simulink model "tutorial4"  (R2020a)
settings: Solver=FixedStepAuto  StartTime=0.0  StopTime=10.0  FixedStep=1e-3  RelTol=1e-3  EnableMultiTasking=on
libraries: dspstat3 x2
settings Model: ExtModeTrigDuration=5  Creator=qasim  LastModifiedBy=qasim
settings OptimizationCC: EnhancedBackFolding=on  PassReuseOutputArgsAs=Individual arguments  ZeroExternalMemoryAtStartup=off  ZeroInternalMemoryAtStartup=off  MaxStackSize=64  OptimizeBlockOrder=speed  DifferentSizesBufferReuse=on  OptimizationCustomize=off  EfficientTunableParamExpr=on
settings DebuggingCC: ParameterTunabilityLossMsg=error
settings HardwareCC: ProdBitPerPointer=32  ProdBitPerSizeT=32  ProdBitPerPtrDiffT=32  ProdLargestAtomicInteger=Long  ProdLargestAtomicFloat=Double  ProdWordSize=32  ProdHWDeviceType=ARM Compatible->ARM Cortex
settings SFSimCC: MATLABDynamicMemAlloc=off
settings RTWCC: SystemTargetFile=ert.tlc  HardwareBoard=NXP FRDM-K64F  TemplateMakefile=ert_default_tmf  Toolchain=GNU Tools for ARM Embedded Processors
settings CodeAppCC: ForceParamTrailComments=on  IgnoreCustomStorageClasses=off  OperatorAnnotations=on  SimulinkDataObjDesc=on  SFDataObjDesc=on  InsertBlockDesc=on

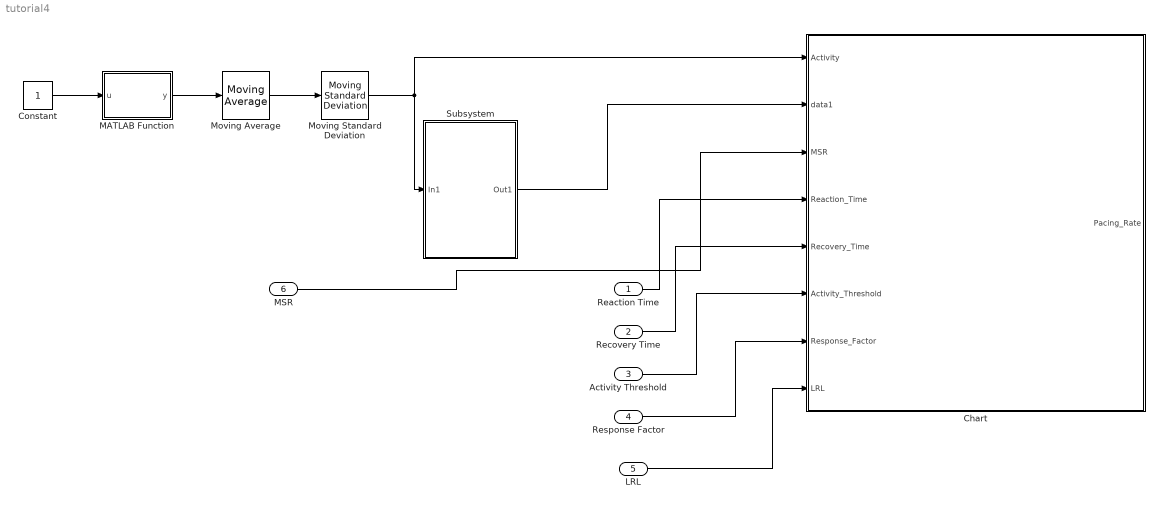
== system tutorial4 ==
  Reaction Time : Inport
  Recovery Time : Inport  Port=2
  Activity Threshold : Inport  Port=3
  Response Factor : Inport  Port=4
  LRL : Inport  Port=5
  MSR : Inport  Port=6
  Chart : Stateflow chart  TreatAsAtomicUnit=on
  Constant : Constant
  MATLAB Function : MATLAB Function  TreatAsAtomicUnit=on
  Moving Average : dspstat3/Moving Average  Method=Sliding window  ForgettingFactorPort=off  SpecifyWindowLength=on  WindowLength=4  ForgettingFactor=0.9  SimulateUsing=Code generation
  Moving Standard Deviation : dspstat3/Moving Standard Deviation  Method=Sliding window  ForgettingFactorPort=off  SpecifyWindowLength=on  WindowLength=4  ForgettingFactor=0.9  SimulateUsing=Code generation
      settings: SourceProductBaseCode=DS
  Subsystem : Subsystem
  wires:
  Constant/1 -> MATLAB Function/1(u)
  MATLAB Function/1(y) -> Moving Average/1
  Moving Average/1 -> Moving Standard Deviation/1
  Moving Standard Deviation/1 -> Subsystem/1(In1), Chart/1(Activity)
  Recovery Time/1 -> Chart/5(Recovery_Time)
  Reaction Time/1 -> Chart/4(Reaction_Time)
  Activity Threshold/1 -> Chart/6(Activity_Threshold)
  Response Factor/1 -> Chart/7(Response_Factor)
  LRL/1 -> Chart/8(LRL)
  Subsystem/1(Out1) -> Chart/2(data1)
  MSR/1 -> Chart/3(MSR)

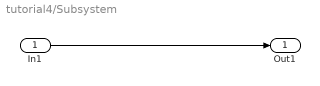
== system tutorial4/Subsystem ==
  In1 : Inport
  Out1 : Outport
  wires:
  In1/1 -> Out1/1

== matlab function tutorial4/MATLAB Function ==
  data: u input; y output
function y = fcn(u)

y = sqrt(u(1)^2+u(2)^2+u(3)^2);

== stateflow chart tutorial4/Chart ==
  state Start
    entry:
    Pacing_Rate = LRL
    Time = 0
  state Increase_Rate
    entry:
    Time = 0
    during:
    Pacing_Rate = Pacing_Rate + LRL
  state Decrease_Rate
    entry:
    Time = 0
    during:
  state Rate_above_LRL
    entry:
    Pacing_Rate = MSR
  state Rate_below_LRL
    entry:
    Pacing_Rate = LRL
  (default) -> Start [order 1]
  Start -> Increase_Rate [order 1] : [Activity <= Activity_Thresholf]
  Start -> Decrease_Rate [order 2] : [Activity > Activity_Threshold]
  Increase_Rate -> Increase_Rate
  Decrease_Rate -> Decrease_Rate
  (default) -> Decrease_Rate [order 2] : [Activity > Activity_Threshold]
  (default) -> Increase_Rate [order 3] : [Activity <= Activity_Threshold]
  (default) -> Decrease_Rate [order 7]
  (default) -> Rate_above_LRL [order 4] : [Pacing_Rate >= MSR]
  (default) -> Rate_below_LRL [order 5] : [Pacing_Rate < LRL]
  (default) -> Increase_Rate [order 6]
  data: Activity input; data1 input; MSR input; Reaction_Time input; Recovery_Time input; Activity_Threshold input; Response_Factor input; LRL input; Pacing_Rate output; Time local
